simulink model "Sliding_mode_O"  (R2017a)
settings: Solver=VariableStepAuto  StartTime=0.0  StopTime=4  RelTol=1e-3
values from neighbouring files (symbols this model uses):
  l1 = 5    [Non_linear_observers_.m]
  l2 = 3    [Non_linear_observers_.m]
settings Model: Creator=firass2019  LastModifiedBy=firass2019

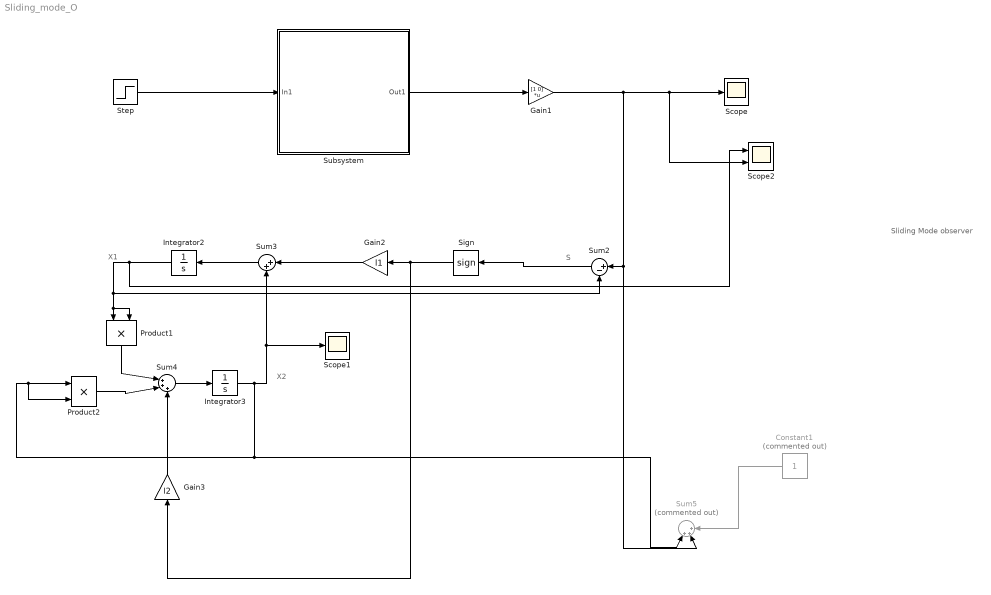
== system Sliding_mode_O ==
  note: Sliding Mode observer
  note: X2
  note: X1
  note: S
  Constant1 : Constant  Commented=on
  Gain1 : Gain  Gain=[1 0]  Multiplication=Matrix(K*u)
  Gain2 : Gain  Gain=l1
  Gain3 : Gain  Gain=l2
  Integrator2 : Integrator
  Integrator3 : Integrator
  Product1 : Product
  Product2 : Product
  Scope : Scope
  Scope1 : Scope
  Scope2 : Scope  NumInputPorts=2
  Sign : Signum  ZeroCross=off
  Step : Step  Time=0  After=0  SampleTime=0
  Subsystem : Subsystem
  Sum2 : Sum  Inputs=|+-
  Sum3 : Sum  Inputs=|++
  Sum4 : Sum  Inputs=|+++
  Sum5 : Sum  Commented=on  Inputs=|+++
  wires:
  Step/1 -> Subsystem/1(In1)
  Subsystem/1(Out1) -> Gain1/1
  Gain1/1 -> Sum5/2, Sum2/1, Scope2/2, Scope/1
  Sum2/1 -> Sign/1
  Sign/1 -> Gain3/1, Gain2/1
  Gain2/1 -> Sum3/1
  Integrator3/1 -> Sum5/1, Product2/2, Product2/1, Scope1/1, Sum3/2
  Sum3/1 -> Integrator2/1
  Integrator2/1 -> Scope2/1, Sum2/2, Product1/2, Product1/1
  Product1/1 -> Sum4/1
  Product2/1 -> Sum4/2
  Sum4/1 -> Integrator3/1
  Constant1/1 -> Sum5/3
  Gain3/1 -> Sum4/3

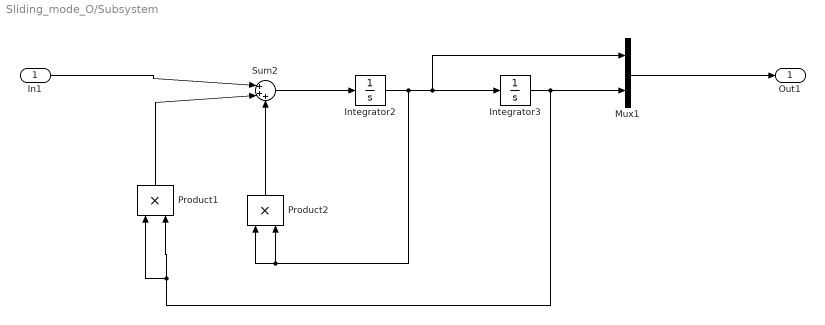
== system Sliding_mode_O/Subsystem ==
  In1 : Inport
  Integrator2 : Integrator  InitialCondition=0.1
  Integrator3 : Integrator
  Mux1 : Mux  Inputs=2
  Product1 : Product
  Product2 : Product
  Sum2 : Sum  Inputs=|+++
  Out1 : Outport
  wires:
  In1/1 -> Sum2/1
  Mux1/1 -> Out1/1
  Integrator2/1 -> Product2/1, Product2/2, Mux1/1, Integrator3/1
  Integrator3/1 -> Mux1/2, Product1/2, Product1/1
  Sum2/1 -> Integrator2/1
  Product1/1 -> Sum2/2
  Product2/1 -> Sum2/3
